simulink model "ADC_Capture_4x4_IQ_DDR4"  (R2019b)
settings: Solver=FixedStepDiscrete  StartTime=0.0  StopTime=inf  RelTol=1e-3
InitFcn:
  | init_ADC_Capture_4x4_IQ_DDR4
values from neighbouring files (symbols this model uses):
  Fs = ConverterSamplingRate/DDC_DUC_factor    (= 512000000)    [init_ADC_Capture_4x4_IQ_DDR4.m]
  N = 14    [init_ADC_Capture_4x4_IQ_DDR4.m]
  sim_CaptureLength = CaptureLength    (= 4096)    [init_ADC_Capture_4x4_IQ_DDR4.m]
  sim_RdFrameSize = 64    [init_ADC_Capture_4x4_IQ_DDR4.m]
  sim_RdNumFrames = ceil(sim_CaptureLength/sim_RdFrameSize)    [init_ADC_Capture_4x4_IQ_DDR4.m]
undefined symbols (not defined in the file or in its folder): config, DDR, Fo
libraries: hdlsllib x35, simulink x20, ddr4_behavioral_mdl x1, AXIDMALib x1, dsphdlsigops x1
(part 1 of 3)
Description:
  | GenericDesign_AX4Master
  | 
  | Template model for GenericDesign ADC/DAC inports/outports with master/slave DMA connection and AXI4 Master
settings Model: DataTypeOverride=Off  Creator=darenlee  LastModifiedBy=ajtro
settings DataIOCC: SaveFormat=StructureWithTime  SaveOutput=off  InspectSignalLogs=on  SaveTime=off  ReturnWorkspaceOutputs=off
settings OptimizationCC: BlockReduction=off  ConditionallyExecuteInputs=off  DefaultParameterBehavior=Inlined
settings DebuggingCC: AlgebraicLoopMsg=error  SingleTaskRateTransMsg=error
settings HardwareCC: ProdBitPerPointer=32  ProdBitPerSizeT=32  ProdBitPerPtrDiffT=32  ProdLargestAtomicFloat=None  ProdIntDivRoundTo=Undefined  ProdEndianess=Unspecified  ProdWordSize=32  ProdHWDeviceType=ASIC/FPGA->ASIC/FPGA  TargetBitPerPointer=64  TargetBitPerSizeT=64  TargetBitPerPtrDiffT=64  TargetLongLongMode=on  TargetIntDivRoundTo=Zero  TargetEndianess=LittleEndian  TargetWordSize=64  TargetHWDeviceType=Custom Processor->MATLAB Host Computer  ProdEqTarget=off
settings SFSimCC: CustomCodeUndefinedFunction=UseInterfaceOnly

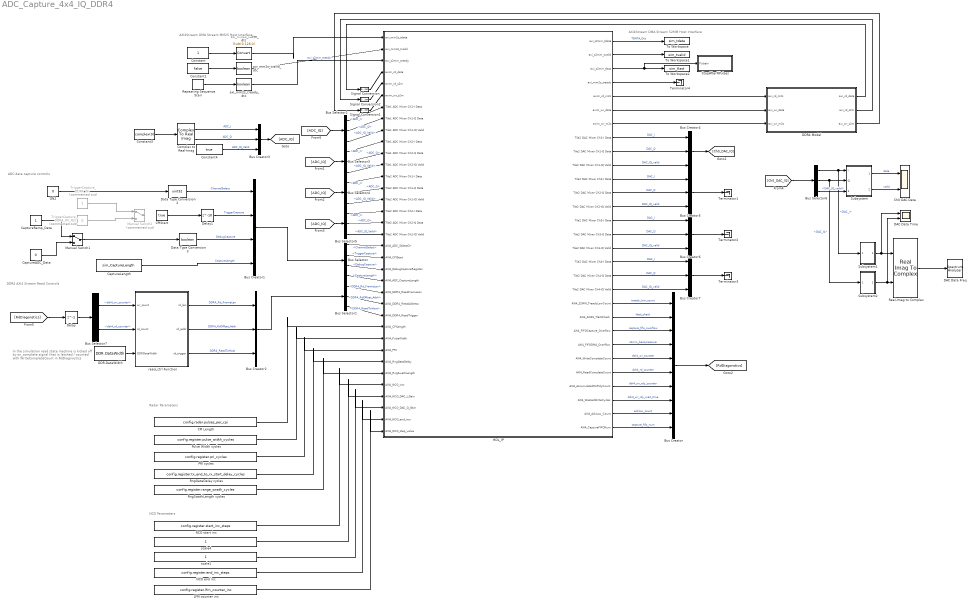
== system ADC_Capture_4x4_IQ_DDR4 ==
  note: Radar Parameters
  note: AXI4Stream DMA Stream S2MM Host Interface
  note: AXI4Stream DMA Stream MM2S Host Interface
  note: In the simulation read state machine
      | is kicked off by wr_complete signal that
      | is latched / counted with WriteCompleteCount
      | in RdDiagnostics
  note: DDR4 AXI4 Stream Read Controls
  note: ADC data capture controls
  note: NCO Parameters
  Bus Creator : BusCreator  Inputs=10
  Bus Creator1 : BusCreator  Inputs=4
  Bus Creator{2..7} (6 alike) : BusCreator  Inputs=3
  Bus Selector : BusSelector  OutputSignals=ChannelSelect,TriggerCapture,DebugCapture,CaptureLength
  Bus Selector1 : BusSelector  OutputSignals=DDR4_Rd_FrameLen,DDR4_RdOffset_Addr,DDR4_ReadToHost
  Bus Selector{2..5} (4 alike) : BusSelector  OutputSignals=ADC_I,ADC_Q,ADC_IQ_Valid
  Bus Selector6 : BusSelector  OutputSignals=DAC_I,DAC_Q,DAC_IQ_valid
  Bus Selector7 : BusSelector  OutputSignals=ddr4_wr_counter,ddr4_rd_counter
  CPI Length : Constant  Value=config.radar.pulses_per_cpi  OutDataTypeStr=uint32  SampleTime=-1
  CPIStart : Constant  Value=true  OutDataTypeStr=boolean  SampleTime=-1
  CaptureADC_Data : Constant  Value=0  OutDataTypeStr=boolean  SampleTime=-1
  CaptureLength : Constant  Value=sim_CaptureLength  OutDataTypeStr=uint32  SampleTime=-1
  CaptureRamp_Data : Constant  OutDataTypeStr=boolean  SampleTime=-1
  Ch0 DAC Data : Scope  NumInputPorts=2
  Complex to Real-Imag : ComplexToRealImag
  Constant : Constant  SampleTime=-1
  Constant1 : Constant  Value=false  SampleTime=-1
  Constant3 : Constant  Value=complex(0)  OutDataTypeStr=uint64  SampleTime=1
  Constant4 : Constant  Value=true  SampleTime=-1
  DAC Data Freq : SpectrumAnalyzer
  DAC Data Time : Scope  NumInputPorts=2
  DDR.DataWidth : Constant  Value=DDR.DataWidth
  DDR4 Model : Subsystem
  Data Type Conversion2 : DataTypeConversion  OutDataTypeStr=uint32
  Data Type Conversion3 : DataTypeConversion  OutDataTypeStr=boolean
  Delay : Delay  DelayLength=1
  Delay1 : Delay  DelayLength=10
  HDL_IP : Subsystem  TreatAsAtomicUnit=on
  LFM counter inc : Constant  Value=config.register.lfm_counter_inc  OutDataTypeStr=int32  SampleTime=-1
  Manual Switch1 : ManualSwitch
  Manual Switch2 : ManualSwitch  Commented=on
  NCO end inc : Constant  Value=config.register.end_inc_steps  OutDataTypeStr=int32  SampleTime=-1
  NCO start inc : Constant  Value=config.register.start_inc_steps  OutDataTypeStr=int32  SampleTime=-1
  ON2 : Constant  Value=0  OutDataTypeStr=uint32  SampleTime=-1
  PRI cycles : Constant  Value=config.register.pri_cycles  OutDataTypeStr=uint32  SampleTime=-1
  Pulse Width cycles : Constant  Value=config.register.pulse_width_cycles  OutDataTypeStr=uint32  SampleTime=-1
  Real-Imag to Complex : RealImagToComplex
  Repeating Sequence Stair : simulink/Sources/Repeating Sequence Stair  OutValues=[0 0 1 1 1 1 1 1 1 1 1];  tsamp=1  OutMin=[]  OutMax=[]  OutDataTypeStr=double  OutputDataTypeScalingMode=double  OutDataType=fixdt(0,8)  ConRadixGroup=Best Precision: Vector-wise  OutScaling=2^-12
      settings: AttributesFormatString=---------------\nIpr = 0\nOpr = 0
  RngGateDelay cycles : Constant  Value=config.register.tx_end_to_rx_start_delay_cycles  OutDataTypeStr=uint32  SampleTime=-1
  RngSwathLength cycles : Constant  Value=config.register.range_swath_cycles  OutDataTypeStr=uint32  SampleTime=-1
  Signal Conversion : SignalConversion  OverrideOpt=off
  Signal Conversion1 : SignalConversion  OverrideOpt=off
  Signal Conversion2 : SignalConversion  OverrideOpt=off
  StopAfterNPulses : Subsystem  mask{MaxPulse=sim_RdNumFrames, DelayTerm=100}
      mask prompts: MaxPulse "Max Pulses"; DelayTerm "Delay after pulse counter"
      mask Display: disp('Sim Terminate')
  Subsystem : Subsystem
  Subsystem1 : Subsystem
  Subsystem2 : Subsystem
  Terminator{1..4} (4 alike) : Terminator
  To Workspace : ToWorkspace  VariableName=sim_tdata  SampleTime=-1
      settings: Save2DSignal=2-D array (concatenate along first dimension)
  To Workspace1 : ToWorkspace  VariableName=sim_tvalid  SampleTime=-1
      settings: Save2DSignal=2-D array (concatenate along first dimension)
  To Workspace2 : ToWorkspace  VariableName=sim_tlast  SampleTime=-1
      settings: Save2DSignal=2-D array (concatenate along first dimension)
  TriggerCapture_DDR4_Wr : Constant  Commented=on  OutDataTypeStr=boolean  SampleTime=-1
  TriggerCapture_DDR4_Wr_Rst : Constant  Commented=on  Value=0  OutDataTypeStr=boolean  SampleTime=-1
  axi_mm2s_tdata_dtc : DataTypeConversion  OutDataTypeStr=fixdt(0,128,0)
  axi_mm2s_tready_dtc : DataTypeConversion  OutDataTypeStr=boolean
  axi_mm2s_tvalid_dtc : DataTypeConversion  OutDataTypeStr=boolean
  read_ctrl Function : MATLAB Function  TreatAsAtomicUnit=on
  scale1 : Constant  OutDataTypeStr=fixdt(0,8,7)  SampleTime=-1
  scale4 : Constant  OutDataTypeStr=fixdt(0,8,7)  SampleTime=-1
  wires:
  CaptureADC_Data/1 -> Manual Switch1/2
  CaptureRamp_Data/1 -> Manual Switch1/1
  Constant3/1 -> Complex to Real-Imag/1
  read_ctrl Function/2(rd_addr) -> Bus Creator2/2  "DDR4_RdOffset_Addr"
  TriggerCapture_DDR4_Wr_Rst/1 -> Manual Switch2/2
  read_ctrl Function/1(rd_len) -> Bus Creator2/1  "DDR4_Rd_FrameLen"
  Constant/1 -> axi_mm2s_tdata_dtc/1
  Manual Switch1/1 -> Data Type Conversion3/1
  CaptureLength/1 -> Bus Creator1/4  "CaptureLength"
  TriggerCapture_DDR4_Wr/1 -> Manual Switch2/1
  CPIStart/1 -> Delay1/1
  Data Type Conversion2/1 -> Bus Creator1/1  "ChannelSelect"
  ON2/1 -> Data Type Conversion2/1
  HDL_IP/8(Tile2 DAC Mixer Ch1-I Data) -> Bus Creator4/1  "DAC_I"
  axi_mm2s_tready_dtc/1 -> HDL_IP/3(axi_s2mm_tready)  "axi_s2mm_tready"
  HDL_IP/19(Tile2 DAC Mixer Ch4-IQ Valid) -> Bus Creator7/3  "DAC_IQ_valid"
  axi_mm2s_tdata_dtc/1 -> HDL_IP/1(axi_mm2s_tdata)
  axi_mm2s_tvalid_dtc/1 -> HDL_IP/2(axi_mm2s_tvalid)
  HDL_IP/2(axi_s2mm_tvalid) -> To Workspace1/1
  HDL_IP/7(axim_wr_m2s) -> DDR4 Model/3(axi_wr_m2s)
  HDL_IP/1(axi_s2mm_tdata) -> To Workspace/1  "TDATA_Out"
  Constant1/1 -> axi_mm2s_tvalid_dtc/1
  HDL_IP/5(axim_rd_m2s) -> DDR4 Model/1(axi_rd_m2s)
  Repeating Sequence Stair/1 -> axi_mm2s_tready_dtc/1
  DDR4 Model/3("axi_wr_s2m ") -> Signal Conversion1/1
  DDR4 Model/2("axi_rd_s2m ") -> Signal Conversion2/1
  HDL_IP/9(Tile2 DAC Mixer Ch1-Q Data) -> Bus Creator4/2  "DAC_Q"
  HDL_IP/17(Tile2 DAC Mixer Ch4-I Data) -> Bus Creator7/1  "DAC_I"
  HDL_IP/18(Tile2 DAC Mixer Ch4-Q Data) -> Bus Creator7/2  "DAC_Q"
  HDL_IP/10(Tile2 DAC Mixer Ch1-IQ Valid) -> Bus Creator4/3  "DAC_IQ_valid"
  Complex to Real-Imag/2 -> Bus Creator3/2  "ADC_Q"
  HDL_IP/20(AXI4_S2MM_TreadyLowCount) -> Bus Creator/1  "tready_low_count"
  HDL_IP/21(AXI4_AXI4S_TlastCheck) -> Bus Creator/2  "tlast_check"
  HDL_IP/22(AXI4_FIFOCapture_Overflow) -> Bus Creator/3  "capture_fifo_overflow"
  HDL_IP/3(axi_s2mm_tlast) -> StopAfterNPulses/1(PulseIn), To Workspace2/1
  HDL_IP/23(AXI4_FIFODMA_Overflow) -> Bus Creator/4  "s2mm_backpressure"
  HDL_IP/24(AXI4_WriteCompleteCount) -> Bus Creator/5  "ddr4_wr_counter"
  HDL_IP/25(AXI4_ReadCompleteCount) -> Bus Creator/6  "ddr4_rd_counter"
  HDL_IP/26(AXI4_AccumulatedWrRdyCount) -> Bus Creator/7  "ddr4_wr_rdy_counter"
  HDL_IP/27(AXI4_WastedWriteCycles) -> Bus Creator/8  "ddr4_wr_rdy_wait_time"
  HDL_IP/28(AXI4_AckLow_Count) -> Bus Creator/9  "acklow_count"
  HDL_IP/29(AXI4_CaptureFIFONum) -> Bus Creator/10  "capture_fifo_num"
  Bus Creator/1 -> [RdDiagonstics]
  HDL_IP/6(axim_wr_data) -> DDR4 Model/2(axi_wr_data)
  DDR4 Model/1(axi_rd_data) -> Signal Conversion/1
  Delay1/1 -> Bus Creator1/2  "TriggerCapture"
  Data Type Conversion3/1 -> Bus Creator1/3  "DebugCapture"
  Bus Creator1/1 -> Bus Selector/1
  Bus Selector/1 -> HDL_IP/19(AXI4_ADC_SelectCh)  "<ChannelSelect>"
  Bus Selector/2 -> HDL_IP/20(AXI4_CPIStart)  "<TriggerCapture>"
  Bus Selector/3 -> HDL_IP/21(AXI4_DebugCaptureRegister)  "<DebugCapture>"
  Bus Selector/4 -> HDL_IP/22(AXI4_ADC_CaptureLength)  "<CaptureLength>"
  Bus Creator2/1 -> Bus Selector1/1
  Bus Selector1/3 -> HDL_IP/25(AXI4_DDR4_ReadTrigger)  "<DDR4_ReadToHost>"
  Bus Selector1/2 -> HDL_IP/24(AXI4_DDR4_ReadAddress)  "<DDR4_RdOffset_Addr>"
  Bus Selector1/1 -> HDL_IP/23(AXI4_DDR4_ReadFrameLen)  "<DDR4_Rd_FrameLen>"
  Signal Conversion/1 -> HDL_IP/4(axim_rd_data)
  Signal Conversion1/1 -> HDL_IP/6(axim_wr_s2m)
  Signal Conversion2/1 -> HDL_IP/5(axim_rd_s2m)
  Complex to Real-Imag/1 -> Bus Creator3/1  "ADC_I"
  Constant4/1 -> Bus Creator3/3  "ADC_IQ_Valid"
  Bus Creator3/1 -> [ADC_IQ]
  [ADC_IQ] -> Bus Selector2/1
  Bus Selector2/1 -> HDL_IP/7(Tile1 ADC Mixer Ch1-I Data)  "<ADC_I>"
  Bus Selector3/3 -> HDL_IP/12(Tile1 ADC Mixer Ch2-IQ Valid)  "<ADC_IQ_Valid>"
  [ADC_IQ] -> Bus Selector3/1
  Bus Selector3/1 -> HDL_IP/10(Tile1 ADC Mixer Ch2-I Data)  "<ADC_I>"
  Bus Selector3/2 -> HDL_IP/11(Tile1 ADC Mixer Ch2-Q Data)  "<ADC_Q>"
  Bus Selector4/3 -> HDL_IP/15(Tile2 ADC Mixer Ch1-IQ Valid)  "<ADC_IQ_Valid>"
  [ADC_IQ] -> Bus Selector4/1
  Bus Selector4/1 -> HDL_IP/13(Tile2 ADC Mixer Ch1-I Data)  "<ADC_I>"
  Bus Selector4/2 -> HDL_IP/14(Tile2 ADC Mixer Ch1-Q Data)  "<ADC_Q>"
  Bus Selector5/3 -> HDL_IP/18(Tile2 ADC Mixer Ch2-IQ Valid)  "<ADC_IQ_Valid>"
  [ADC_IQ] -> Bus Selector5/1
  Bus Selector5/1 -> HDL_IP/16(Tile2 ADC Mixer Ch2-I Data)  "<ADC_I>"
  Bus Selector5/2 -> HDL_IP/17(Tile2 ADC Mixer Ch2-Q Data)  "<ADC_Q>"
  Subsystem/1(IQ_Data) -> Ch0 DAC Data/1  "data"
  Bus Creator4/1 -> [Ch0_DAC_IQ]
  [Ch0_DAC_IQ] -> Bus Selector6/1
  Subsystem/2(ValidOut) -> Ch0 DAC Data/2  "valid"
  Bus Selector6/1 -> Subsystem1/1(In1), Subsystem/1(I)  "<DAC_I>"
  Bus Selector6/2 -> Subsystem2/1(In1), Subsystem/2(Q)  "<DAC_Q>"
  Bus Selector6/3 -> Subsystem/3(ValidIn)  "<DAC_IQ_valid>"
  HDL_IP/11(Tile2 DAC Mixer Ch2-I Data) -> Bus Creator5/1  "DAC_I"
  HDL_IP/12(Tile2 DAC Mixer Ch2-Q Data) -> Bus Creator5/2  "DAC_Q"
  HDL_IP/13(Tile2 DAC Mixer Ch2-IQ Valid) -> Bus Creator5/3  "DAC_IQ_valid"
  Bus Creator5/1 -> Terminator1/1
  HDL_IP/14(Tile2 DAC Mixer Ch3-I Data) -> Bus Creator6/1  "DAC_I"
  HDL_IP/15(Tile2 DAC Mixer Ch3-Q Data) -> Bus Creator6/2  "DAC_Q"
  HDL_IP/16(Tile2 DAC Mixer Ch3-IQ Valid) -> Bus Creator6/3  "DAC_IQ_valid"
  Bus Creator6/1 -> Terminator2/1
  Bus Creator7/1 -> Terminator3/1
  HDL_IP/4(axi_mm2s_tready) -> Terminator4/1
  [RdDiagonstics] -> Delay/1
  read_ctrl Function/3(rd_trigger) -> Bus Creator2/3  "DDR4_ReadToHost"
  Bus Selector7/1 -> read_ctrl Function/1(wr_count)  "<ddr4_wr_counter>"
  Bus Selector7/2 -> read_ctrl Function/2(rd_count)  "<ddr4_rd_counter>"
  Delay/1 -> Bus Selector7/1
  CPI Length/1 -> HDL_IP/26(AXI4_CPILength)
  Pulse Width cycles/1 -> HDL_IP/27(AXI4_PulseWidth)
  PRI cycles/1 -> HDL_IP/28(AXI4_PRI)
  RngGateDelay cycles/1 -> HDL_IP/29(AXI4_RngGateDelay)
  LFM counter inc/1 -> HDL_IP/35(AXI4_NCO_step_value)
  NCO end inc/1 -> HDL_IP/34(AXI4_NCO_end_incr)
  NCO start inc/1 -> HDL_IP/31(AXI4_NCO_incr)
  scale4/1 -> HDL_IP/32(AXI4_NCO_DAC_I_Gain)
  scale1/1 -> HDL_IP/33(AXI4_NCO_DAC_Q_Gain)
  RngSwathLength cycles/1 -> HDL_IP/30(AXI4_RngSwathLength)
  Subsystem2/1(Out1) -> Real-Imag to Complex/2, DAC Data Time/2
  Subsystem1/1(Out1) -> Real-Imag to Complex/1, DAC Data Time/1
  Real-Imag to Complex/1 -> DAC Data Freq/1
  Bus Selector2/2 -> HDL_IP/8(Tile1 ADC Mixer Ch1-Q Data)  "<ADC_Q>"
  Bus Selector2/3 -> HDL_IP/9(Tile1 ADC Mixer Ch1-IQ Valid)  "<ADC_IQ_Valid>"
  DDR.DataWidth/1 -> read_ctrl Function/3(DDRDataWidth)

== system ADC_Capture_4x4_IQ_DDR4/DDR4 Model ==
  axi_rd_m2s : Inport
  axi_wr_data : Inport  Port=2
  axi_wr_m2s : Inport  Port=3
  DDR : ddr4_behavioral_mdl/DDR  DDR3_DEPTH=DDR.Depth  WR_RD_DATAWIDTH=DDR.DataWidth  INIT_DDR3=off  INIT_ADDR=0  INIT_DATA=DDR.InitData  OutDataTypeStr=DDR.DataType  READY_DUTY_CYL=1  toggle=off
  DDR3 : Subsystem  Commented=on  mask{DDR3_DEPTH=1024, WR_RD_DATAWIDTH=128, INIT_DDR3=on, INIT_ADDR=0, INIT_DATA=fi(zeros(1,1024),0,128,0), OutDataTypeStr=fixdt(0,128,0), READY_DUTY_CYL=1, toggle=off}
      mask prompts: DDR3_DEPTH "DDR3 DEPTH"; WR_RD_DATAWIDTH "DDR Data Width"; INIT_DDR3 "Initialize DDR3"; INIT_ADDR "DDR3 Initial Address"; INIT_DATA "DDR3 Initialization data"; OutDataTypeStr "Simulink:blkprm_prompts:UNIFIEDDATATYPE"; READY_DUTY_CYL "READY Duty Cycle"; toggle "Read Valid Toggling"
      mask help: DDR3 Simulation model
      mask init:
      | if(DDR3_DEPTH<=1)
      |     error('DDR size should be greater than 1' )  
      | end
      | 
      | if(READY_DUTY_CYL>1)
      |   error('should be less than 1' )  
      | end
      |    
      | 
      | %%Initialization Value
      | if(INIT_DDR3==true)
      |     if(isempty(INIT_ADDR))
      |      error('Enter Initial address' )  
      |     end   
      | end
      mask TypeOptions WR_RD_DATAWIDTH: 32 | 64 | 128
      mask Callback INIT_DDR3:
      | % Get the mask parameter values. This is a cell
      | %   array of character vectors.
      | maskStr = get_param(gcb,'INIT_DDR3');
      | 
      | % The pop-up menu is the first mask parameter.
      | %   Check the value selected in the pop-up
      | if strcmp(maskStr,'on')
      | 
      |     % Set the visibility of both parameters on when
      |     %   User-defined is selected in the pop-up.
      | 
      |     set_param(gcb,'MaskEnables',{'on','on','on','on','on','on','on','on'});
      | 
      | else
      | 
      |     % Turn off the visibility of the Value field
      |     %   when User-defined is not selected.
      | 
      |     set_param(gcb,'MaskEnables',{'on','on','on','off','off','on','on','on'});
      | 
      |     % Set the character vector in the Values field equal to the
      |     % character vector selected in the Gain pop-up menu.
      | 
      |     %maskStr{2}=maskStr{1};
      | 
      | end
      mask TypeOptions OutDataTypeStr: axi_wr_data/OutDataTypeStr | axi_rd_data/OutDataTypeStr
      mask DialogControl DescGroupVar Prompt: DDR
      mask DialogControl DDR3_INIT Prompt: DDR3 Initialization
      mask DialogControl PARAM_GROUP Prompt: DDR3 Initialization Parameters
      mask DialogControl OutDataTypeStr Prompt: Data type:
      mask DialogControl READY_DUTY_CYL Tooltip: between 0 to 1
  Terminator : Terminator
  axi_rd_data : Outport
  "axi_rd_s2m " : Outport  Port=2
  "axi_wr_s2m " : Outport  Port=3
  wires:
  DDR/4 -> "axi_wr_s2m "/1
  DDR/2 -> axi_rd_data/1
  axi_rd_m2s/1 -> DDR/1
  axi_wr_data/1 -> DDR/2
  DDR/3 -> "axi_rd_s2m "/1
  axi_wr_m2s/1 -> DDR/3
  DDR/1 -> Terminator/1

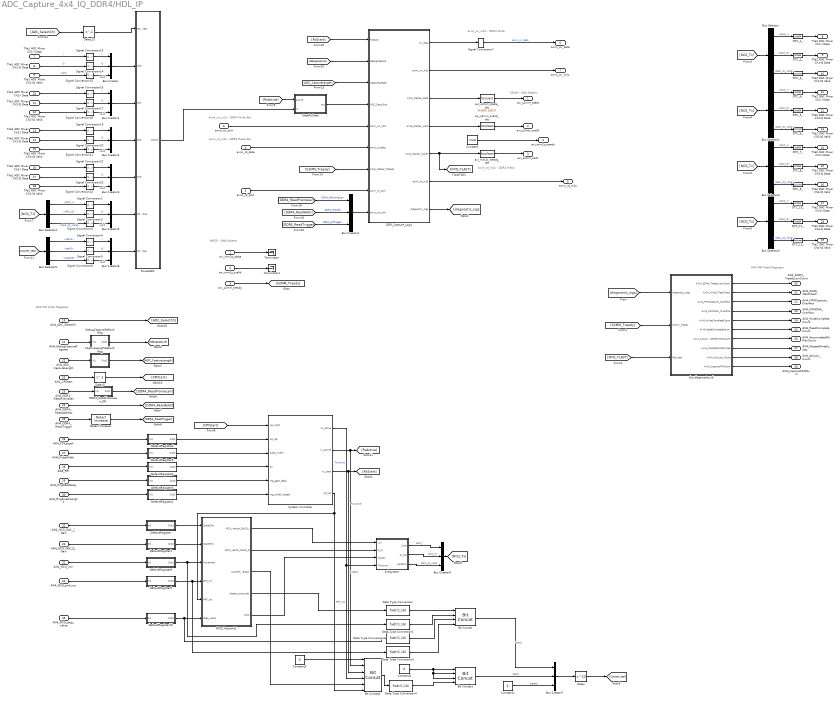
== system ADC_Capture_4x4_IQ_DDR4/HDL_IP ==
  note: MM2S - DMA Stream
  note: axim_wr_m2s - DDR4 Write
  note: axim_rd_m2s - DDR4 Read Ack
  note: axim_rd_m2s - DDR4 Read
  note: axim_wr_m2s - DDR4 Write Ack
  note: S2MM - DMA Stream
  note: AXI4 MM Write Registers
  note: AXI4 MM Read Registers
  axi_mm2s_tdata : Inport
  axi_mm2s_tvalid : Inport  Port=2
  axi_s2mm_tready : Inport  Port=3
  axim_rd_data : Inport  Port=4
  axim_rd_s2m : Inport  Port=5
  axim_wr_s2m : Inport  Port=6
  Tile1 ADC Mixer Ch1-I Data : Inport  Port=7  OutDataTypeStr=uint64
  Tile1 ADC Mixer Ch1-Q Data : Inport  Port=8  OutDataTypeStr=uint64
  Tile1 ADC Mixer Ch1-IQ Valid : Inport  Port=9  OutDataTypeStr=boolean
  Tile1 ADC Mixer Ch2-I Data : Inport  Port=10  OutDataTypeStr=uint64
  Tile1 ADC Mixer Ch2-Q Data : Inport  Port=11  OutDataTypeStr=uint64
  Tile1 ADC Mixer Ch2-IQ Valid : Inport  Port=12  OutDataTypeStr=boolean
  Tile2 ADC Mixer Ch1-I Data : Inport  Port=13  OutDataTypeStr=uint64
  Tile2 ADC Mixer Ch1-Q Data : Inport  Port=14  OutDataTypeStr=uint64
  Tile2 ADC Mixer Ch1-IQ Valid : Inport  Port=15  OutDataTypeStr=boolean
  Tile2 ADC Mixer Ch2-I Data : Inport  Port=16  OutDataTypeStr=uint64
  Tile2 ADC Mixer Ch2-Q Data : Inport  Port=17  OutDataTypeStr=uint64
  Tile2 ADC Mixer Ch2-IQ Valid : Inport  Port=18  OutDataTypeStr=boolean
  AXI4_ADC_SelectCh : Inport  Port=19
  AXI4_CPIStart : Inport  Port=20
  AXI4_DebugCaptureRegister : Inport  Port=21
  AXI4_ADC_CaptureLength : Inport  Port=22
  AXI4_DDR4_ReadFrameLen : Inport  Port=23
  AXI4_DDR4_ReadAddress : Inport  Port=24
  AXI4_DDR4_ReadTrigger : Inport  Port=25
  AXI4_CPILength : Inport  Port=26
  AXI4_PulseWidth : Inport  Port=27
  AXI4_PRI : Inport  Port=28
  AXI4_RngGateDelay : Inport  Port=29
  AXI4_RngSwathLength : Inport  Port=30
  AXI4_NCO_incr : Inport  Port=31
  AXI4_NCO_DAC_I_Gain : Inport  Port=32
  AXI4_NCO_DAC_Q_Gain : Inport  Port=33
  AXI4_NCO_end_incr : Inport  Port=34
  AXI4_NCO_step_value : Inport  Port=35
  Bit Concat : hdlsllib/Logic and Bit Operations/Bit Concat  numInputs=4
      settings: SourceProductName=Simulink
  Bit Concat1 : hdlsllib/Logic and Bit Operations/Bit Concat  numInputs=4
      settings: SourceProductName=Simulink
  Bit Concat2 : hdlsllib/Logic and Bit Operations/Bit Concat  numInputs=6
      settings: SourceProductName=Simulink
  Bus Creator{,1..8} (9 alike) : BusCreator  Inputs=3
  Bus Selector{,1..4} (5 alike) : BusSelector  OutputSignals=DAC_I,DAC_Q,DAC_IQ_Valid
  Bus Selector5 : BusSelector  OutputSignals=test1,test2,signal3
  "CaptureLengthDefaultReg " : Subsystem
  Constant : Constant  Value=true  SampleTime=-1
  Constant1 : Constant  OutDataTypeStr=boolean
  Constant2 : Constant  Value=0  OutDataTypeStr=fixdt(1,16)
  Constant3 : Constant  Value=0  OutDataTypeStr=fixdt(1,11)  SampleTime=-1
  DDR4_ReadFrameLen_DR : Subsystem
  DDR_Capture_Logic : Subsystem
  DTC_10_ : DataTypeConversion  OutDataTypeStr=uint64  ConvertRealWorld=Stored Integer (SI)
  DTC_11_ : DataTypeConversion  OutDataTypeStr=uint64  ConvertRealWorld=Stored Integer (SI)
  DTC_12_ : DataTypeConversion  OutDataTypeStr=boolean  ConvertRealWorld=Stored Integer (SI)
  DTC_1_ : DataTypeConversion  OutDataTypeStr=uint64  ConvertRealWorld=Stored Integer (SI)
  DTC_2_ : DataTypeConversion  OutDataTypeStr=uint64  ConvertRealWorld=Stored Integer (SI)
  DTC_3_ : DataTypeConversion  OutDataTypeStr=boolean  ConvertRealWorld=Stored Integer (SI)
  DTC_4_ : DataTypeConversion  OutDataTypeStr=uint64  ConvertRealWorld=Stored Integer (SI)
  DTC_5_ : DataTypeConversion  OutDataTypeStr=uint64  ConvertRealWorld=Stored Integer (SI)
  DTC_6_ : DataTypeConversion  OutDataTypeStr=boolean  ConvertRealWorld=Stored Integer (SI)
  DTC_7_ : DataTypeConversion  OutDataTypeStr=uint64  ConvertRealWorld=Stored Integer (SI)
  DTC_8_ : DataTypeConversion  OutDataTypeStr=uint64  ConvertRealWorld=Stored Integer (SI)
  DTC_9_ : DataTypeConversion  OutDataTypeStr=boolean  ConvertRealWorld=Stored Integer (SI)
  Data Type Conversion{,1..4} (5 alike) : DataTypeConversion  OutMin=-32768  OutMax=32767  OutDataTypeStr=fixdt(1,16)
  DebugCaptureDefaultReg : Subsystem
  DefaultRegister : Subsystem
  DefaultRegister1 : Subsystem
  DefaultRegister10 : Subsystem
  DefaultRegister2 : Subsystem
  DefaultRegister3 : Subsystem
  DefaultRegister4 : Subsystem
  DefaultRegister5 : Subsystem
  DefaultRegister6 : Subsystem
  DefaultRegister8 : Subsystem
  DefaultRegister9 : Subsystem
  Delay : Delay  DelayLength=10
  Delay13 : Delay  DelayLength=1
  Delay5 : Delay  DelayLength=1
  Detect Increase : simulink/Logic and Bit Operations/Detect Increase  vinit=0.0  OutDataTypeStr=boolean
  GateRxData : Subsystem
      settings: PortSchema="{\"entries\":[{\"content\":{\"sides\":[{\"content\":{\"connectorIds\":[\"In1\",\"In2\"]},\"type\":\"ConnectorPlacement.EquallySpacedRectSide\",\"uuid\":\"73340317-26ec-445b-a38a-ecaac9c95ad8\"},{\"content\":{\"connectorIds\":[\"Out1\"],\"side\":\"RIGHT\"},\"type\":\"ConnectorPlacement.EquallySpacedRectSide\",\"uuid\":\"4d52f90a-d813-4789-957e-2a9657680730\"},{\"content\":{\"connectorIds\":[],\"side\":\"TOP\"},\"type\":\"ConnectorPlacement.EquallySpacedRectSide\",\"uuid\":\"fb82458e-1347-4e0b-94aa-c00767c75e11\"}]},\"type\":\"ConnectorPlacement.EquallySpacedConnector\",\"uuid\":\"ddf0ba30-d999-4968-8664-a134857b39f1\"}],\"packageUris\":[\"http://schema.mathworks.com/mf0/Connector/19700101\"],\"version\":\"1.0\"}"
  NCO_Transmit1 : Subsystem
  RouteADC : Subsystem
  Signal Conversion{1..7,13..24} (19 alike) : SignalConversion  OverrideOpt=off
  Subsystem : Subsystem
  System Controller : MATLAB Function  TreatAsAtomicUnit=on
  Terminator : Terminator
  Terminator1 : Terminator
  axi_mm2s_tready_dtc : DataTypeConversion  OutDataTypeStr=boolean
  axi_s2mm_tdata_dtc : DataTypeConversion  OutDataTypeStr=fixdt(0,128,0)
  axi_s2mm_tvalid_dtc : DataTypeConversion  OutDataTypeStr=boolean
  dut_diagnostics_rd : Subsystem
  axi_s2mm_tdata : Outport  VectorParamsAs1DForOutWhenUnconnected=off
  axi_s2mm_tvalid : Outport  Port=2  VectorParamsAs1DForOutWhenUnconnected=off
  axi_s2mm_tlast : Outport  Port=3
  axi_mm2s_tready : Outport  Port=4  VectorParamsAs1DForOutWhenUnconnected=off
  axim_rd_m2s : Outport  Port=5  VectorParamsAs1DForOutWhenUnconnected=off
  axim_wr_data : Outport  Port=6  VectorParamsAs1DForOutWhenUnconnected=off
  axim_wr_m2s : Outport  Port=7  VectorParamsAs1DForOutWhenUnconnected=off
  Tile2 DAC Mixer Ch1-I Data : Outport  Port=8  OutDataTypeStr=uint64
  Tile2 DAC Mixer Ch1-Q Data : Outport  Port=9  OutDataTypeStr=uint64
  Tile2 DAC Mixer Ch1-IQ Valid : Outport  Port=10  OutDataTypeStr=boolean
  Tile2 DAC Mixer Ch2-I Data : Outport  Port=11  OutDataTypeStr=uint64
  Tile2 DAC Mixer Ch2-Q Data : Outport  Port=12  OutDataTypeStr=uint64
  Tile2 DAC Mixer Ch2-IQ Valid : Outport  Port=13  OutDataTypeStr=boolean
  Tile2 DAC Mixer Ch3-I Data : Outport  Port=14  OutDataTypeStr=uint64
  Tile2 DAC Mixer Ch3-Q Data : Outport  Port=15  OutDataTypeStr=uint64
  Tile2 DAC Mixer Ch3-IQ Valid : Outport  Port=16  OutDataTypeStr=boolean
  Tile2 DAC Mixer Ch4-I Data : Outport  Port=17  OutDataTypeStr=uint64
  Tile2 DAC Mixer Ch4-Q Data : Outport  Port=18  OutDataTypeStr=uint64
  Tile2 DAC Mixer Ch4-IQ Valid : Outport  Port=19  OutDataTypeStr=boolean
  AXI4_S2MM_TreadyLowCount : Outport  Port=20  VectorParamsAs1DForOutWhenUnconnected=off
  AXI4_AXI4S_TlastCheck : Outport  Port=21  VectorParamsAs1DForOutWhenUnconnected=off
  AXI4_FIFOCapture_Overflow : Outport  Port=22  VectorParamsAs1DForOutWhenUnconnected=off
  AXI4_FIFODMA_Overflow : Outport  Port=23  VectorParamsAs1DForOutWhenUnconnected=off
  AXI4_WriteCompleteCount : Outport  Port=24  VectorParamsAs1DForOutWhenUnconnected=off
  AXI4_ReadCompleteCount : Outport  Port=25  VectorParamsAs1DForOutWhenUnconnected=off
  AXI4_AccumulatedWrRdyCount : Outport  Port=26  VectorParamsAs1DForOutWhenUnconnected=off
  AXI4_WastedWriteCycles : Outport  Port=27  VectorParamsAs1DForOutWhenUnconnected=off
  AXI4_AckLow_Count : Outport  Port=28  VectorParamsAs1DForOutWhenUnconnected=off
  AXI4_CaptureFIFONum : Outport  Port=29  VectorParamsAs1DForOutWhenUnconnected=off
  wires:
  axi_mm2s_tdata/1 -> Terminator/1
  axi_mm2s_tvalid/1 -> Terminator1/1
  axi_s2mm_tready/1 -> [S2MM_Tready]
  DDR_Capture_Logic/3(AXIS_Master_Data) -> axi_s2mm_tdata_dtc/1
  DDR_Capture_Logic/4(AXIS_Master_Valid) -> axi_s2mm_tvalid_dtc/1
  DDR_Capture_Logic/5(AXIS_Master_TLAST) -> [FIFO_TLAST], axi_mm2s_tready_dtc/1
  axi_s2mm_tdata_dtc/1 -> axi_s2mm_tdata/1
  axi_s2mm_tvalid_dtc/1 -> axi_s2mm_tvalid/1
  axi_mm2s_tready_dtc/1 -> axi_s2mm_tlast/1
  DDR_Capture_Logic/2(axim_wr_m2s) -> axim_wr_m2s/1
  DDR_Capture_Logic/1(wr_data) -> Signal Conversion7/1
  DDR_Capture_Logic/6(axim_rd_m2s) -> axim_rd_m2s/1
  Signal Conversion7/1 -> axim_wr_data/1  "axim_wr_data"
  axim_wr_s2m/1 -> DDR_Capture_Logic/5(axim_wr_s2m)
  Tile1 ADC Mixer Ch1-I Data/1 -> Signal Conversion13/1  "I"
  Tile1 ADC Mixer Ch1-IQ Valid/1 -> Signal Conversion15/1  "Valid"
  Tile1 ADC Mixer Ch2-I Data/1 -> Signal Conversion16/1
  Tile1 ADC Mixer Ch2-Q Data/1 -> Signal Conversion17/1
  Tile1 ADC Mixer Ch2-IQ Valid/1 -> Signal Conversion18/1
  Tile2 ADC Mixer Ch1-I Data/1 -> Signal Conversion19/1
  Tile2 ADC Mixer Ch1-Q Data/1 -> Signal Conversion20/1
  Tile2 ADC Mixer Ch1-IQ Valid/1 -> Signal Conversion21/1
  Bus Selector/1 -> DTC_1_/1  "<DAC_I>"
  DTC_1_/1 -> Tile2 DAC Mixer Ch1-I Data/1
  Bus Selector/2 -> DTC_2_/1  "<DAC_Q>"
  DTC_2_/1 -> Tile2 DAC Mixer Ch1-Q Data/1
  Bus Selector/3 -> DTC_3_/1  "<DAC_IQ_Valid>"
  DTC_3_/1 -> Tile2 DAC Mixer Ch1-IQ Valid/1
  Bus Selector1/1 -> DTC_4_/1  "<DAC_I>"
  DTC_4_/1 -> Tile2 DAC Mixer Ch2-I Data/1
  Bus Selector1/2 -> DTC_5_/1  "<DAC_Q>"
  DTC_5_/1 -> Tile2 DAC Mixer Ch2-Q Data/1
  Bus Selector1/3 -> DTC_6_/1  "<DAC_IQ_Valid>"
  DTC_6_/1 -> Tile2 DAC Mixer Ch2-IQ Valid/1
  Bus Selector2/1 -> DTC_7_/1  "<DAC_I>"
  DTC_7_/1 -> Tile2 DAC Mixer Ch3-I Data/1
  Bus Selector2/2 -> DTC_8_/1  "<DAC_Q>"
  DTC_8_/1 -> Tile2 DAC Mixer Ch3-Q Data/1
  Bus Selector2/3 -> DTC_9_/1  "<DAC_IQ_Valid>"
  DTC_9_/1 -> Tile2 DAC Mixer Ch3-IQ Valid/1
  Bus Selector3/1 -> DTC_10_/1  "<DAC_I>"
  DTC_10_/1 -> Tile2 DAC Mixer Ch4-I Data/1
  Bus Selector3/2 -> DTC_11_/1  "<DAC_Q>"
  DTC_11_/1 -> Tile2 DAC Mixer Ch4-Q Data/1
  Bus Selector3/3 -> DTC_12_/1  "<DAC_IQ_Valid>"
  DTC_12_/1 -> Tile2 DAC Mixer Ch4-IQ Valid/1
  Tile1 ADC Mixer Ch1-Q Data/1 -> Signal Conversion14/1  "Q"
  Signal Conversion13/1 -> Bus Creator/1  "I"
  Signal Conversion14/1 -> Bus Creator/2  "Q"
  Signal Conversion15/1 -> Bus Creator/3  "Valid"
  Bus Creator/1 -> RouteADC/2(Ch0)
  Signal Conversion18/1 -> Bus Creator1/3  "Valid"
  Signal Conversion16/1 -> Bus Creator1/1  "I"
  Signal Conversion17/1 -> Bus Creator1/2  "Q"
  Bus Creator1/1 -> RouteADC/3(Ch1)
  Signal Conversion19/1 -> Bus Creator2/1  "I"
  Signal Conversion20/1 -> Bus Creator2/2  "Q"
  Signal Conversion21/1 -> Bus Creator2/3  "Valid"
  Bus Creator2/1 -> RouteADC/4(Ch2)
  Tile2 ADC Mixer Ch2-Q Data/1 -> Signal Conversion23/1
  Signal Conversion24/1 -> Bus Creator3/3  "Valid"
  Signal Conversion23/1 -> Bus Creator3/2  "Q"
  Signal Conversion22/1 -> Bus Creator3/1  "I"
  Tile2 ADC Mixer Ch2-I Data/1 -> Signal Conversion22/1
  Tile2 ADC Mixer Ch2-IQ Valid/1 -> Signal Conversion24/1
  Bus Creator3/1 -> RouteADC/5(Ch3)
  Delay13/1 -> RouteADC/1(PortSelect)
  [RxStart] -> DDR_Capture_Logic/1(RxStart)
  [DebugCapture] -> DDR_Capture_Logic/2(DebugCapture)
  [ADC_CaptureLength] -> DDR_Capture_Logic/3(CaptureLength)
  axim_rd_s2m/1 -> DDR_Capture_Logic/8(axim_rd_s2m)
  [S2MM_Tready] -> DDR_Capture_Logic/7(AXIS_Master_TReady)
  [DDR4_ReadTrigger] -> Bus Creator4/3  "DDR4_RdTrigger"
  [DDR4_ReadFrameLen] -> Bus Creator4/1  "DDR4_RdFrameLen"
  [DDR4_ReadAddr] -> Bus Creator4/2  "DDR4_RdAddr"
  Bus Creator4/1 -> DDR_Capture_Logic/9(axim_rd_cmd)
  DebugCaptureDefaultReg/1(Out1) -> [DebugCapture]
  AXI4_DebugCaptureRegister/1 -> DebugCaptureDefaultReg/1(In1)
  AXI4_CPIStart/1 -> Delay5/1
  AXI4_ADC_CaptureLength/1 -> "CaptureLengthDefaultReg "/1(In1)
  "CaptureLengthDefaultReg "/1(Out1) -> [ADC_CaptureLength]
  Detect Increase/1 -> [DDR4_ReadTrigger]
  AXI4_DDR4_ReadTrigger/1 -> Detect Increase/1
  AXI4_DDR4_ReadAddress/1 -> [DDR4_ReadAddr]
  AXI4_DDR4_ReadFrameLen/1 -> DDR4_ReadFrameLen_DR/1(In1)
  DDR4_ReadFrameLen_DR/1(Out1) -> [DDR4_ReadFrameLen]
  DDR_Capture_Logic/7(diagonstic_sigs) -> [diagnostic_sigs]
  [diagnostic_sigs] -> dut_diagnostics_rd/1(diagnostic_sigs)
  [S2MM_Tready] -> dut_diagnostics_rd/2(s2mm_tready)
  [FIFO_TLAST] -> dut_diagnostics_rd/3(fifo_tlast)
  dut_diagnostics_rd/10(AXI4_CaptureFIFONum) -> AXI4_CaptureFIFONum/1
  dut_diagnostics_rd/3(AXI4_FIFOCapture_Overflow) -> AXI4_FIFOCapture_Overflow/1
  dut_diagnostics_rd/6(AXI4_ReadCompleteCount) -> AXI4_ReadCompleteCount/1
  dut_diagnostics_rd/7(AXI4_AccumulatedWrRdyCount) -> AXI4_AccumulatedWrRdyCount/1
  dut_diagnostics_rd/9(AXI4_AckLow_Count) -> AXI4_AckLow_Count/1
  dut_diagnostics_rd/2(AXI4_AXI4S_TlastCheck) -> AXI4_AXI4S_TlastCheck/1
  dut_diagnostics_rd/4(AXI4_FIFODMA_Overflow) -> AXI4_FIFODMA_Overflow/1
  dut_diagnostics_rd/8(AXI4_WastedWriteCycles) -> AXI4_WastedWriteCycles/1
  dut_diagnostics_rd/5(AXI4_WriteCompleteCount) -> AXI4_WriteCompleteCount/1
  dut_diagnostics_rd/1(AXI4_S2MM_TreadyLowCount) -> AXI4_S2MM_TreadyLowCount/1
  axim_rd_data/1 -> DDR_Capture_Logic/6(axim_rd_data)
  [NCO_Tx] -> Bus Selector/1
  [NCO_Tx] -> Bus Selector1/1
  [NCO_Tx] -> Bus Selector2/1
  [NCO_Tx] -> Bus Selector3/1
  Constant/1 -> axi_mm2s_tready/1
  System Controller/3(rx_start) -> Bit Concat2/3, [RxStart]  "RxStart"
  Delay5/1 -> [CPIStart]
  [CPIStart] -> System Controller/1(cpi_start)
  AXI4_CPILength/1 -> DefaultRegister6/1(In1)
  AXI4_PulseWidth/1 -> DefaultRegister5/1(In1)
  System Controller/2(rx_active) -> Bit Concat2/2, [RxActive]  "RxActive"
  GateRxData/1(out) -> DDR_Capture_Logic/4(ADC_Data_Bus)
  [RxActive] -> GateRxData/1(active)
  RouteADC/1(ChOut) -> GateRxData/2(in)
  System Controller/1(tx_active) -> Bit Concat2/4, Subsystem/4(TxActive)  "TxActive"
  AXI4_PRI/1 -> DefaultRegister4/1(In1)
  AXI4_RngGateDelay/1 -> DefaultRegister3/1(In1)
  AXI4_ADC_SelectCh/1 -> [ADC_SelectCh]
  [ADC_SelectCh] -> Delay13/1
  DefaultRegister/1(Out2) -> NCO_Transmit1/1(ScaleCh0)
  AXI4_NCO_DAC_I_Gain/1 -> DefaultRegister/1(In1)
  DefaultRegister1/1(Out2) -> NCO_Transmit1/2(ScaleCh1)
  AXI4_NCO_DAC_Q_Gain/1 -> DefaultRegister1/1(In1)
  DefaultRegister10/1(Out2) -> Data Type Conversion2/1, NCO_Transmit1/6(Step_value)
  DefaultRegister8/1(Out2) -> Data Type Conversion1/1, NCO_Transmit1/3(Increment)
  AXI4_NCO_incr/1 -> DefaultRegister8/1(In1)
  AXI4_NCO_end_incr/1 -> DefaultRegister9/1(In1)
  AXI4_NCO_step_value/1 -> DefaultRegister10/1(In1)
  DefaultRegister9/1(Out2) -> Data Type Conversion3/1, NCO_Transmit1/4(End_inc)
  NCO_Transmit1/2(NCO_Vector_DAC0_Q) -> Subsystem/2(Q_in)
  NCO_Transmit1/1(NCO_Vector_DAC0_I) -> Subsystem/1(I_in)
  System Controller/4(prf_rst) -> Bit Concat2/6, NCO_Transmit1/5(PRF_rst)  "PRF_rst"
  Subsystem/1(I_out) -> Bus Creator6/1  "DAC_I"
  Subsystem/2(Q_out) -> Bus Creator6/2  "DAC_Q"
  Subsystem/3(ValidOut) -> Bus Creator6/3  "DAC_IQ_Valid"
  Bus Creator6/1 -> [NCO_Tx]
  AXI4_RngSwathLength/1 -> DefaultRegister2/1(In1)
  DefaultRegister2/1(Out2) -> System Controller/6(rng_swath_length)
  DefaultRegister3/1(Out2) -> System Controller/5(rng_gate_delay)
  DefaultRegister4/1(Out2) -> System Controller/4(pri)
  DefaultRegister5/1(Out2) -> System Controller/3(pulse_width)
  DefaultRegister6/1(Out2) -> System Controller/2(cpi_len)
  Signal Conversion1/1 -> Bus Creator5/1  "I"
  Signal Conversion2/1 -> Bus Creator5/2  "Q"
  Bus Creator5/1 -> RouteADC/6(DACDebug)
  Signal Conversion3/1 -> Bus Creator5/3  "Valid"
  Bus Selector4/2 -> Signal Conversion2/1  "<DAC_Q>"
  Bus Selector4/3 -> Signal Conversion3/1  "<DAC_IQ_Valid>"
  Bus Selector4/1 -> Signal Conversion1/1  "<DAC_I>"
  [NCO_Tx] -> Bus Selector4/1
  Constant1/1 -> Bus Creator7/3  "signal3"
  Bus Creator7/1 -> Delay/1
  Bus Selector5/2 -> Signal Conversion5/1  "<test2>"
  Bus Creator8/1 -> RouteADC/7(CounterDebug)
  Signal Conversion4/1 -> Bus Creator8/1  "I"
  Signal Conversion5/1 -> Bus Creator8/2  "Q"
  Bus Selector5/3 -> Signal Conversion6/1  "<signal3>"
  Signal Conversion6/1 -> Bus Creator8/3  "Valid"
  Bus Selector5/1 -> Signal Conversion4/1  "<test1>"
  [Counter_test] -> Bus Selector5/1
  Delay/1 -> [Counter_test]
  Bit Concat2/1 -> Data Type Conversion4/1
  Data Type Conversion4/1 -> Bit Concat1/4
  Data Type Conversion3/1 -> Bit Concat/4
  Data Type Conversion1/1 -> Bit Concat/2
  Data Type Conversion2/1 -> Bit Concat/3
  Constant2/1 -> Bit Concat1/3, Bit Concat1/2, Bit Concat1/1
  Bit Concat1/1 -> Bus Creator7/2  "test2"
  Bit Concat/1 -> Bus Creator7/1  "test1"
  Data Type Conversion/1 -> Bit Concat/1
  NCO_Transmit1/4(phase_count_dot) -> Data Type Conversion/1
  Constant3/1 -> Bit Concat2/1
  NCO_Transmit1/5("Valid ") -> Subsystem/3(ValidIn)
  NCO_Transmit1/3("Counter_reload ") -> Bit Concat2/5

== system ADC_Capture_4x4_IQ_DDR4/StopAfterNPulses ==
  PulseIn : Inport
  Add : Sum  AccumDataTypeStr=uint32
  Compare To Constant1 : simulink/Logic and Bit Operations/Compare To Constant  relop===  const=MaxPulse  OutDataTypeStr=boolean
  Data Type Conversion : DataTypeConversion  OutDataTypeStr=uint32
  Delay1 : Delay  DelayLength=DelayTerm
  Delay2 : Delay  DelayLength=1
  Stop Simulation : Stop
  wires:
  PulseIn/1 -> Data Type Conversion/1
  Data Type Conversion/1 -> Add/1
  Add/1 -> Delay2/1
  Delay2/1 -> Compare To Constant1/1, Add/2
  Compare To Constant1/1 -> Delay1/1
  Delay1/1 -> Stop Simulation/1

== system ADC_Capture_4x4_IQ_DDR4/Subsystem ==
  I : Inport
  Q : Inport  Port=2
  ValidIn : Inport  Port=3
  Format_I : Subsystem
  Format_Q : Subsystem
  Real-Imag to Complex : RealImagToComplex
  IQ_Data : Outport
  ValidOut : Outport  Port=2
  wires:
  Format_Q/1(Out1) -> Real-Imag to Complex/2
  Real-Imag to Complex/1 -> IQ_Data/1
  Format_I/1(Out1) -> Real-Imag to Complex/1
  I/1 -> Format_I/1(In1)
  Q/1 -> Format_Q/1(In1)
  ValidIn/1 -> ValidOut/1

== system ADC_Capture_4x4_IQ_DDR4/Subsystem1 ==
  In1 : Inport
  Bit Slice : hdlsllib/Logic and Bit Operations/Bit Slice  lidx=47  ridx=32
  Bit Slice2 : hdlsllib/Logic and Bit Operations/Bit Slice  lidx=63  ridx=48
  Bit Slice3 : hdlsllib/Logic and Bit Operations/Bit Slice  lidx=31  ridx=16
  Bit Slice5 : hdlsllib/Logic and Bit Operations/Bit Slice  lidx=15  ridx=0
  Data Type Conversion{,1..3} (4 alike) : DataTypeConversion  OutDataTypeStr=fixdt(1,16,0)  ConvertRealWorld=Stored Integer (SI)
  Vector Concatenate : Concatenate  NumInputs=4  Mode=Multidimensional array
  Out1 : Outport  VectorParamsAs1DForOutWhenUnconnected=off
  wires:
  Vector Concatenate/1 -> Out1/1
  Data Type Conversion/1 -> Vector Concatenate/1
  Bit Slice5/1 -> Data Type Conversion/1
  Bit Slice/1 -> Data Type Conversion2/1
  Data Type Conversion1/1 -> Vector Concatenate/2
  In1/1 -> Bit Slice/1, Bit Slice2/1, Bit Slice3/1, Bit Slice5/1
  Data Type Conversion3/1 -> Vector Concatenate/4
  Bit Slice2/1 -> Data Type Conversion3/1
  Bit Slice3/1 -> Data Type Conversion1/1
  Data Type Conversion2/1 -> Vector Concatenate/3

== system ADC_Capture_4x4_IQ_DDR4/Subsystem2 ==
  In1 : Inport
  Bit Slice : hdlsllib/Logic and Bit Operations/Bit Slice  lidx=47  ridx=32
  Bit Slice2 : hdlsllib/Logic and Bit Operations/Bit Slice  lidx=63  ridx=48
  Bit Slice3 : hdlsllib/Logic and Bit Operations/Bit Slice  lidx=31  ridx=16
  Bit Slice5 : hdlsllib/Logic and Bit Operations/Bit Slice  lidx=15  ridx=0
  Data Type Conversion{,1..3} (4 alike) : DataTypeConversion  OutDataTypeStr=fixdt(1,16,0)  ConvertRealWorld=Stored Integer (SI)
  Vector Concatenate : Concatenate  NumInputs=4  Mode=Multidimensional array
  Out1 : Outport  VectorParamsAs1DForOutWhenUnconnected=off
  wires:
  Vector Concatenate/1 -> Out1/1
  Data Type Conversion/1 -> Vector Concatenate/1
  Bit Slice5/1 -> Data Type Conversion/1
  Bit Slice/1 -> Data Type Conversion2/1
  Data Type Conversion1/1 -> Vector Concatenate/2
  In1/1 -> Bit Slice/1, Bit Slice2/1, Bit Slice3/1, Bit Slice5/1
  Data Type Conversion3/1 -> Vector Concatenate/4
  Bit Slice2/1 -> Data Type Conversion3/1
  Bit Slice3/1 -> Data Type Conversion1/1
  Data Type Conversion2/1 -> Vector Concatenate/3

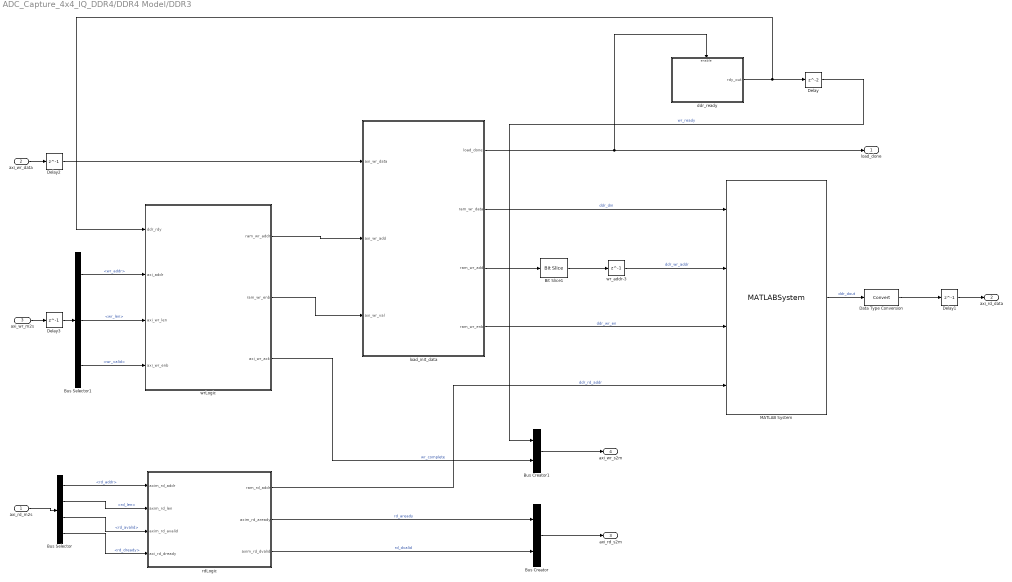
== system ADC_Capture_4x4_IQ_DDR4/DDR4 Model/DDR3 ==
  axi_rd_m2s : Inport
  axi_wr_data : Inport  Port=2  OutDataTypeStr=fixdt(0,128,0)
  axi_wr_m2s : Inport  Port=3
  Bit Slice1 : hdlsllib/Logic and Bit Operations/Bit Slice  lidx=15  ridx=0
  Bus Creator : BusCreator  Inputs=2
  Bus Creator1 : BusCreator  Inputs=2
  Bus Selector : BusSelector  OutputSignals=rd_addr,rd_len,rd_avalid,rd_dready
  Bus Selector1 : BusSelector  OutputSignals=wr_addr,wr_len,wr_valid
  Data Type Conversion : DataTypeConversion
  Delay : Delay
  Delay1 : Delay  DelayLength=1
  Delay2 : Delay  DelayLength=1
  Delay3 : Delay  DelayLength=1
  MATLAB System : MATLABSystem  System=hdl.RAM  RAMType=Simple dual port  WriteOutputValue=New data  RAMInitialValue=0  SimulateUsing=Code generation
      mask Type: hdl.RAM
      mask Display:
      | disp(['Simple' char(10) 'Dual Port' char(10) 'RAM']);
      | port_label('input',1,'din');
      | port_label('input',2,'wr_addr');
      | port_label('input',3,'wr_en');
      | port_label('input',4,'rd_addr');
      | port_label('output',1,'rd_dout');
  ddr_ready : Subsystem
  load_init_data : MATLAB Function  TreatAsAtomicUnit=on
  rdLogic : Subsystem
  wrLogic : Subsystem
  wr_addr-3 : Delay  DelayLength=1
  load_done : Outport  VectorParamsAs1DForOutWhenUnconnected=off
  axi_rd_data : Outport  Port=2  OutDataTypeStr=fixdt(0,128,0)  VectorParamsAs1DForOutWhenUnconnected=off
  axi_rd_s2m : Outport  Port=3  VectorParamsAs1DForOutWhenUnconnected=off
  axi_wr_s2m : Outport  Port=4  VectorParamsAs1DForOutWhenUnconnected=off
  wires:
  Bit Slice1/1 -> wr_addr-3/1
  Delay1/1 -> axi_rd_data/1
  load_init_data/4(ram_wr_enb) -> MATLAB System/3  "ddr_wr_en"
  load_init_data/3(ram_wr_add) -> Bit Slice1/1
  load_init_data/1(load_done) -> ddr_ready/Enable, load_done/1
  MATLAB System/1 -> Data Type Conversion/1  "ddr_dout"
  rdLogic/1(ram_rd_addr) -> MATLAB System/4  "ddr_rd_addr"
  wrLogic/1(ram_wr_addr) -> load_init_data/2(axi_wr_add)
  wrLogic/2(ram_wr_enb) -> load_init_data/3(axi_wr_val)
  wr_addr-3/1 -> MATLAB System/2  "ddr_wr_addr"
  Bus Selector/2 -> rdLogic/2(axim_rd_len)  "<rd_len>"
  Bus Selector/1 -> rdLogic/1(axim_rd_addr)  "<rd_addr>"
  Bus Selector/4 -> rdLogic/4(axi_rd_dready)  "<rd_dready>"
  axi_rd_m2s/1 -> Bus Selector/1
  Bus Selector/3 -> rdLogic/3(axim_rd_avalid)  "<rd_avalid>"
  Bus Selector1/1 -> wrLogic/2(axi_addr)  "<wr_addr>"
  axi_wr_m2s/1 -> Delay3/1
  Bus Selector1/3 -> wrLogic/4(axi_wr_enb)  "<wr_valid>"
  Bus Selector1/2 -> wrLogic/3(axi_wr_len)  "<wr_len>"
  rdLogic/2(axim_rd_aready) -> Bus Creator/1  "rd_aready"
  Bus Creator/1 -> axi_rd_s2m/1
  rdLogic/3(axim_rd_dvalid) -> Bus Creator/2  "rd_dvalid"
  ddr_ready/1(rdy_out) -> Delay/1, wrLogic/1(ddr_rdy)
  Bus Creator1/1 -> axi_wr_s2m/1
  wrLogic/3(axi_wr_ack) -> Bus Creator1/2  "wr_complete"
  Delay/1 -> Bus Creator1/1  "wr_ready"
  load_init_data/2(ram_wr_data) -> MATLAB System/1  "ddr_din"
  axi_wr_data/1 -> Delay2/1
  Delay2/1 -> load_init_data/1(axi_wr_data)
  Delay3/1 -> Bus Selector1/1
  Data Type Conversion/1 -> Delay1/1

== system ADC_Capture_4x4_IQ_DDR4/HDL_IP/CaptureLengthDefaultReg  ==
  In1 : Inport
  Constant3 : Constant  Value=1024  OutDataTypeStr=uint32  SampleTime=-1
  Delay1 : Delay  DelayLength=1
  Switch : Switch  Criteria=u2 ~= 0
  Out1 : Outport  VectorParamsAs1DForOutWhenUnconnected=off
  wires:
  Delay1/1 -> Switch/1, Switch/2
  In1/1 -> Delay1/1
  Constant3/1 -> Switch/3
  Switch/1 -> Out1/1

== system ADC_Capture_4x4_IQ_DDR4/HDL_IP/DDR4_ReadFrameLen_DR ==
  In1 : Inport
  Constant3 : Constant  Value=1024  OutDataTypeStr=uint32  SampleTime=-1
  Delay1 : Delay  DelayLength=1
  Switch : Switch  Criteria=u2 ~= 0
  Out1 : Outport  VectorParamsAs1DForOutWhenUnconnected=off
  wires:
  Delay1/1 -> Switch/1, Switch/2
  In1/1 -> Delay1/1
  Constant3/1 -> Switch/3
  Switch/1 -> Out1/1

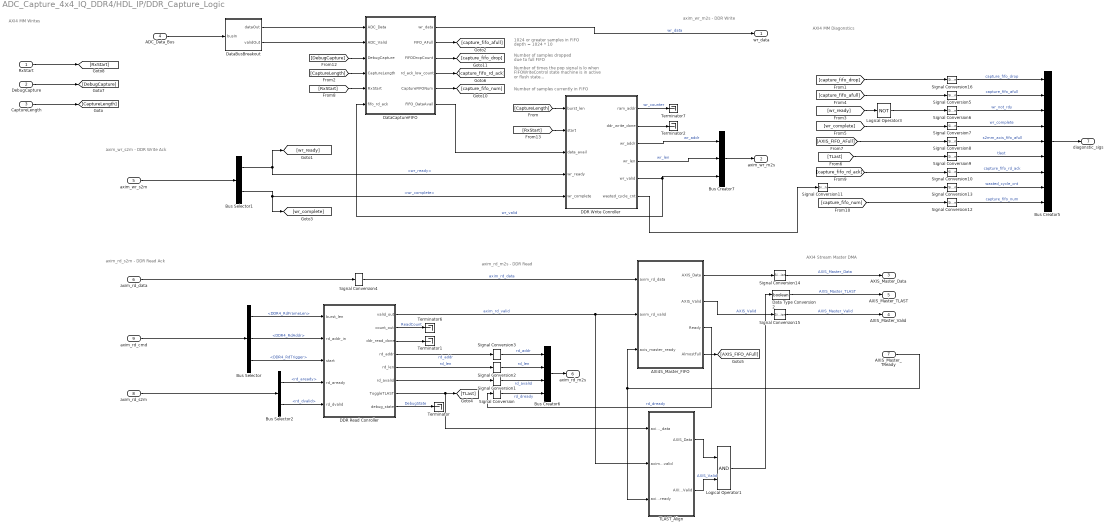
== system ADC_Capture_4x4_IQ_DDR4/HDL_IP/DDR_Capture_Logic ==
  note: 1024 or greater samples in FIFO
      | depth = 1024 * 10
  note: AXI4 MM Writes
  note: AXI4 MM Diagonstics
  note: axim_rd_m2s - DDR Read
  note: AXI4 Stream Master DMA
  note: axim_rd_s2m - DDR Read Ack
  note: axim_wr_m2s - DDR Write
  note: axim_wr_s2m - DDR Write Ack
  note: Number of samples dropped
      | due to full FIFO
  note: Number of times the pop signal is
      | lo when FIFOWriteControl state machine
      | is in active or flush state...
  note: Number of samples currently in FIFO
  RxStart : Inport
  DebugCapture : Inport  Port=2
  CaptureLength : Inport  Port=3
  ADC_Data_Bus : Inport  Port=4
  axim_wr_s2m : Inport  Port=5
  axim_rd_data : Inport  Port=6
  AXIS_Master_TReady : Inport  Port=7
  axim_rd_s2m : Inport  Port=8
  axim_rd_cmd : Inport  Port=9
  "AXI4S_Master_FIFO " : Subsystem
  Bus Creator5 : BusCreator  Inputs=9
  Bus Creator6 : BusCreator  Inputs=4
  Bus Creator7 : BusCreator  Inputs=3
  Bus Selector : BusSelector  OutputSignals=DDR4_RdFrameLen,DDR4_RdAddr,DDR4_RdTrigger
  Bus Selector1 : BusSelector  OutputSignals=wr_ready,wr_complete
  Bus Selector2 : BusSelector  OutputSignals=rd_aready,rd_dvalid
  DDR Read Conroller : MATLAB Function  TreatAsAtomicUnit=on
  DDR Write Conroller : MATLAB Function  TreatAsAtomicUnit=on
  Data Type Conversion2 : DataTypeConversion  OutDataTypeStr=boolean
  DataBusBreakout : Subsystem
  DataCaptureFIFO : Subsystem
  Logical Operator1 : Logic  IconShape=distinctive  AllPortsSameDT=off  OutDataTypeStr=boolean
  Logical Operator3 : Logic  Operator=NOT  IconShape=distinctive  AllPortsSameDT=off  OutDataTypeStr=boolean
  Signal Conversion{,1..16} (17 alike) : SignalConversion  OverrideOpt=off
  TLAST_Align : Subsystem
  Terminator{,1..2,6..7} (5 alike) : Terminator
  wr_data : Outport  VectorParamsAs1DForOutWhenUnconnected=off
  axim_wr_m2s : Outport  Port=2  VectorParamsAs1DForOutWhenUnconnected=off
  AXIS_Master_Data : Outport  Port=3  VectorParamsAs1DForOutWhenUnconnected=off
  AXIS_Master_Valid : Outport  Port=4  VectorParamsAs1DForOutWhenUnconnected=off
  AXIS_Master_TLAST : Outport  Port=5  VectorParamsAs1DForOutWhenUnconnected=off
  axim_rd_m2s : Outport  Port=6  VectorParamsAs1DForOutWhenUnconnected=off
  diagonstic_sigs : Outport  Port=7
  wires:
  "AXI4S_Master_FIFO "/1(AXIS_Data) -> Signal Conversion14/1
  DDR Read Conroller/1(valid_out) -> TLAST_Align/2(axim_rd_valid), "AXI4S_Master_FIFO "/2(axim_rd_valid)  "axim_rd_valid"
  DDR Write Conroller/4(wr_len) -> Bus Creator7/2  "wr_len"
  Bus Selector1/2 -> [wr_complete], DDR Write Conroller/5(wr_complete)  "<wr_complete>"
  DDR Write Conroller/1(ram_addr) -> Terminator7/1  "wr_counter"
  DDR Read Conroller/7(ToggleTLAST) -> [TLast], TLAST_Align/1(axim_rd_data)
  DDR Read Conroller/2(count_out) -> Terminator6/1  "ReadCount"
  Bus Selector/3 -> DDR Read Conroller/3(start)  "<DDR4_RdTrigger>"
  Data Type Conversion2/1 -> AXIS_Master_TLAST/1  "AXIS_Master_TLAST"
  Bus Selector1/1 -> [wr_ready], DDR Write Conroller/4(wr_ready)  "<wr_ready>"
  axim_wr_s2m/1 -> Bus Selector1/1
  DataCaptureFIFO/1(wr_data) -> wr_data/1  "wr_data"
  axim_rd_data/1 -> Signal Conversion4/1
  DDR Read Conroller/5(rd_len) -> Signal Conversion2/1  "rd_len"
  Bus Selector2/2 -> DDR Read Conroller/5(rd_dvalid)  "<rd_dvalid>"
  Bus Selector2/1 -> DDR Read Conroller/4(rd_aready)  "<rd_aready>"
  DDR Read Conroller/6(rd_avalid) -> Signal Conversion1/1
  DDR Read Conroller/4(rd_addr) -> Signal Conversion3/1  "rd_addr"
  DDR Write Conroller/3(wr_addr) -> Bus Creator7/1  "wr_addr"
  [CaptureLength] -> DDR Write Conroller/1(burst_len)
  AXIS_Master_TReady/1 -> TLAST_Align/3(axis_master_ready), "AXI4S_Master_FIFO "/3(axis_master_ready)
  axim_rd_s2m/1 -> Bus Selector2/1
  CaptureLength/1 -> [CaptureLength]
  [CaptureLength] -> DataCaptureFIFO/4(CaptureLength)
  Bus Creator6/1 -> axim_rd_m2s/1
  Bus Creator7/1 -> axim_wr_m2s/1
  DDR Read Conroller/8(debug_state) -> Terminator/1  "DebugState"
  Signal Conversion/1 -> Bus Creator6/4  "rd_dready"
  Signal Conversion1/1 -> Bus Creator6/3  "rd_avalid"
  Signal Conversion2/1 -> Bus Creator6/2  "rd_len"
  Signal Conversion3/1 -> Bus Creator6/1  "rd_addr"
  "AXI4S_Master_FIFO "/3(Ready) -> Signal Conversion/1  "rd_dready"
  "AXI4S_Master_FIFO "/2(AXIS_Valid) -> Signal Conversion15/1  "AXIS_Valid"
  DataCaptureFIFO/2(FIFO_AFull) -> [capture_fifo_afull]
  [capture_fifo_afull] -> Signal Conversion5/1
  [wr_ready] -> Logical Operator3/1
  [TLast] -> Signal Conversion9/1
  "AXI4S_Master_FIFO "/4(AlmostFull) -> [AXIS_FIFO_AFull]
  [AXIS_FIFO_AFull] -> Signal Conversion8/1
  Logical Operator3/1 -> Signal Conversion6/1
  DDR Write Conroller/6(wasted_cycle_cnt) -> Signal Conversion11/1
  RxStart/1 -> [RxStart]
  [RxStart] -> DDR Write Conroller/2(start)
  DebugCapture/1 -> [DebugCapture]
  [DebugCapture] -> DataCaptureFIFO/3(DebugCapture)
  DDR Write Conroller/5(wr_valid) -> Bus Creator7/3, DataCaptureFIFO/6(fifo_rd_ack)  "wr_valid"
  DataCaptureFIFO/6(FIFO_DataAvail) -> DDR Write Conroller/3(data_avail)
  DDR Write Conroller/2(ddr_write_done) -> Terminator2/1
  DataCaptureFIFO/4(rd_ack_low_count) -> [capture_fifo_rd_ack]
  [capture_fifo_rd_ack] -> Signal Conversion10/1
  DataCaptureFIFO/5(CaptureFIFONum) -> [capture_fifo_num]
  [capture_fifo_num] -> Signal Conversion12/1
  axim_rd_cmd/1 -> Bus Selector/1
  Bus Selector/1 -> DDR Read Conroller/1(burst_len)  "<DDR4_RdFrameLen>"
  Bus Selector/2 -> DDR Read Conroller/2(rd_addr_in)  "<DDR4_RdAddr>"
  Signal Conversion4/1 -> "AXI4S_Master_FIFO "/1(axim_rd_data)  "axim_rd_data"
  [wr_complete] -> Signal Conversion7/1
  Signal Conversion11/1 -> Signal Conversion13/1
  Bus Creator5/1 -> diagonstic_sigs/1
  TLAST_Align/2(AXIS_Valid) -> Logical Operator1/2  "AXIS_Valid"
  TLAST_Align/1(AXIS_Data) -> Logical Operator1/1
  Logical Operator1/1 -> Data Type Conversion2/1
  Signal Conversion14/1 -> AXIS_Master_Data/1  "AXIS_Master_Data"
  Signal Conversion15/1 -> AXIS_Master_Valid/1  "AXIS_Master_Valid"
  DataCaptureFIFO/3(FIFODropCount) -> [capture_fifo_drop]
  [capture_fifo_drop] -> Signal Conversion16/1
  Signal Conversion5/1 -> Bus Creator5/2  "capture_fifo_afull"
  Signal Conversion6/1 -> Bus Creator5/3  "wr_not_rdy"
  Signal Conversion7/1 -> Bus Creator5/4  "wr_complete"
  Signal Conversion8/1 -> Bus Creator5/5  "s2mm_axis_fifo_afull"
  Signal Conversion9/1 -> Bus Creator5/6  "tlast"
  Signal Conversion10/1 -> Bus Creator5/7  "capture_fifo_rd_ack"
  Signal Conversion13/1 -> Bus Creator5/8  "wasted_cycle_cnt"
  Signal Conversion12/1 -> Bus Creator5/9  "capture_fifo_num"
  Signal Conversion16/1 -> Bus Creator5/1  "capture_fifo_drop"
  DDR Read Conroller/3(ddr_read_done) -> Terminator1/1
  ADC_Data_Bus/1 -> DataBusBreakout/1(busIn)
  DataBusBreakout/1(dataOut) -> DataCaptureFIFO/1(ADC_Data)
  DataBusBreakout/2(validOut) -> DataCaptureFIFO/2(ADC_Valid)
  [RxStart] -> DataCaptureFIFO/5(RxStart)

== system ADC_Capture_4x4_IQ_DDR4/HDL_IP/DebugCaptureDefaultReg ==
  In1 : Inport
  Delay1 : Delay  DelayLength=1
  Out1 : Outport  VectorParamsAs1DForOutWhenUnconnected=off
  wires:
  In1/1 -> Delay1/1
  Delay1/1 -> Out1/1

== system ADC_Capture_4x4_IQ_DDR4/HDL_IP/DefaultRegister ==
  note: Give it default non-zero value at start-up time
  In1 : Inport
  Compare To Zero : simulink/Logic and Bit Operations/Compare To Zero  relop===  OutDataTypeStr=boolean
  Constant5 : Constant  Value=0.3  OutDataTypeStr=fixdt(0,4,4)  SampleTime=-1
  Delay1 : Delay  DelayLength=1
  Switch2 : Switch  Criteria=u2 > Threshold
  Out2 : Outport  VectorParamsAs1DForOutWhenUnconnected=off
  wires:
  In1/1 -> Delay1/1
  Constant5/1 -> Switch2/1
  Delay1/1 -> Switch2/3, Compare To Zero/1
  Switch2/1 -> Out2/1
  Compare To Zero/1 -> Switch2/2

== system ADC_Capture_4x4_IQ_DDR4/HDL_IP/DefaultRegister1 ==
  note: Give it default non-zero value at start-up time
  In1 : Inport
  Compare To Zero : simulink/Logic and Bit Operations/Compare To Zero  relop===  OutDataTypeStr=boolean
  Constant5 : Constant  Value=0.6  OutDataTypeStr=fixdt(0,4,4)  SampleTime=-1
  Delay1 : Delay  DelayLength=1
  Switch2 : Switch  Criteria=u2 > Threshold
  Out2 : Outport  VectorParamsAs1DForOutWhenUnconnected=off
  wires:
  Compare To Zero/1 -> Switch2/2
  Switch2/1 -> Out2/1
  Delay1/1 -> Compare To Zero/1, Switch2/3
  Constant5/1 -> Switch2/1
  In1/1 -> Delay1/1

== system ADC_Capture_4x4_IQ_DDR4/HDL_IP/DefaultRegister10 ==
  note: Give it default non-zero value at start-up time
  In1 : Inport
  Compare To Zero : simulink/Logic and Bit Operations/Compare To Zero  relop===  OutDataTypeStr=boolean
  Data Type Conversion : DataTypeConversion  OutDataTypeStr=int32
  Delay1 : Delay  DelayLength=1
  Switch2 : Switch  Criteria=u2 > Threshold  OutDataTypeStr=int32
  lfc counter inc : Constant  Value=config.register.lfm_counter_inc  OutDataTypeStr=int32
  Out2 : Outport  VectorParamsAs1DForOutWhenUnconnected=off
  wires:
  lfc counter inc/1 -> Data Type Conversion/1
  In1/1 -> Delay1/1
  Data Type Conversion/1 -> Switch2/1
  Delay1/1 -> Switch2/3, Compare To Zero/1
  Switch2/1 -> Out2/1
  Compare To Zero/1 -> Switch2/2
